simulink model "ImplantationCmd_LQI"  (R2022b)
settings: Solver=FixedStepDiscrete  StartTime=0.0  StopTime=60  FixedStep=Te1  MaxStep=0.001  RelTol=1e-3
values from neighbouring files (symbols this model uses):
  K_lqi = lqr(Apa,Bpa,Q_lqi,R_lqi)    [code.m]
  Kfi = 4.77    [code.m]
  Ki = 5    [code.m]
  Komga = 0.02    [code.m]
  Kteta = 0.875    [code.m]
  r = 0.022    [Validation_param_pend.m]    (also in code.m)
  Te1 = 0.100    (= 0.1)    [code.m]    (also in matlab.mat = 0)
undefined symbols (not defined in the file or in its folder): DiscIntNeverNeededParam, National_Instruments, PCI, pin
libraries: sldrtlib x3, simulink_extras x1
settings Model: SimulationMode=external  ExtModeTrigDuration=60000  Creator=Beauvois  LastModifiedBy=Pedro
settings SolverCC: AlgebraicLoopSolver=TrustRegion
settings DataIOCC: ReturnWorkspaceOutputs=off
settings DebuggingCC: UnconnectedInputMsg=warning  UnconnectedOutputMsg=warning  UnconnectedLineMsg=warning  SFMachineParentedDataDiag=warning  ArithmeticOperatorsInVariantConditions=warning
settings HardwareCC: ProdBitPerLong=64  ProdHWDeviceType=Intel->x86-64 (Linux 64)
settings ModelReferenceCC: EnableRefExpFcnMdlSchedulingChecks=on
settings SFSimCC: SimUseLocalCustomCode=off  CustomCodeUndefinedFunction=UseInterfaceOnly
settings RTWCC: Description=Simulink Desktop Real-Time  SystemTargetFile=sldrt.tlc  TemplateMakefile=sldrt.tmf  RTWUseLocalCustomCode=off  RTWCompilerOptimization=on
settings CodeAppCC: MaxIdLength=95
settings SimulinkDesktopRealTimeCC: TargetLibSuffix=_sldrt.a  TargetPreCompLibLocation=C:\Program Files\MATLAB\R2022b\toolbox\sldrt\lib\win64

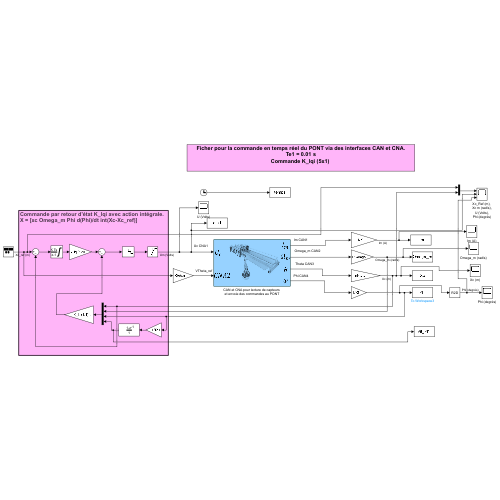
[thumbnail: Simulink's stored preview of the top-level diagram]
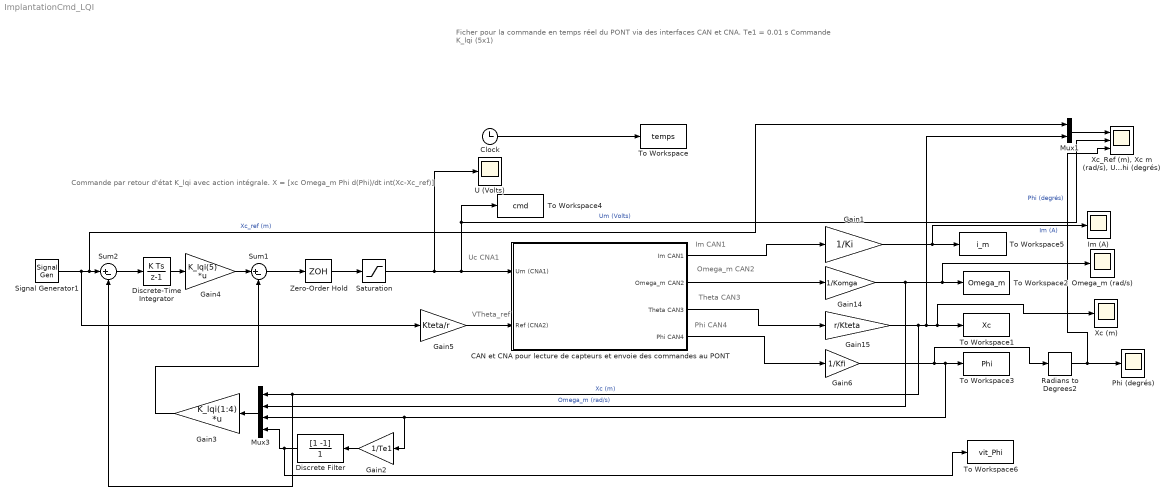
== system ImplantationCmd_LQI ==
  note: Commande par retour d'état K_lqi avec action intégrale.
      | X = [xc Omega_m Phi d(Phi)/dt int(Xc-Xc_ref)]
  note: Im CAN1
  note: Omega_m CAN2
  note: Theta CAN3
  note: Phi CAN4
  note: Uc CNA1
  note: VTheta_ref
  note: Ficher pour la commande en temps réel du PONT via des interfaces CAN et CNA.
      | Te1 = 0.01 s
      | Commande K_lqi (5x1)
  CAN et CNA pour lecture de capteurs et envoie des commandes au PONT : Subsystem
      mask Display: image('$imagefile'); % Use "Edit Image" on toolstrip to change.
  Clock : Clock
  Discrete Filter : DiscreteFilter  Numerator=[1 -1]  Denominator=1  SampleTime=Te1
  Discrete-Time Integrator : DiscreteIntegrator  SampleTime=Te1  LimitOutput=on  UpperSaturationLimit=1  LowerSaturationLimit=-1  ICPrevOutput=DiscIntNeverNeededParam  ICPrevScaledInput=DiscIntNeverNeededParam
  Gain1 : Gain  Gain=1/Ki
  Gain14 : Gain  Gain=1/Komga
  Gain15 : Gain  Gain=r/Kteta
  Gain2 : Gain  Gain=1/Te1
  Gain3 : Gain  Gain=K_lqi(1:4)  Multiplication=Matrix(K*u)
  Gain4 : Gain  Gain=K_lqi(5)  Multiplication=Matrix(K*u)
  Gain5 : Gain  Gain=Kteta/r
  Gain6 : Gain  Gain=1/Kfi
  Im (A) : Scope
  Mux1 : Mux  Inputs=2
  Mux3 : Mux
  Omega_m (rad/s) : Scope
  Phi (degrés) : Scope
  Radians to Degrees2 : simulink_extras/Transformations/Radians to Degrees
  Saturation : Saturate  UpperLimit=9.99  LowerLimit=-9.99
  Signal Generator1 : SignalGenerator  WaveForm=square  Amplitude=0.15  Frequency=0.05
  Sum1 : Sum  Inputs=|+-
  Sum2 : Sum  Inputs=|+-
  To Workspace : ToWorkspace  VariableName=temps  SampleTime=-1
  To Workspace1 : ToWorkspace  VariableName=Xc  SampleTime=-1
  To Workspace2 : ToWorkspace  VariableName=Omega_m  SampleTime=-1
  To Workspace3 : ToWorkspace  VariableName=Phi  SampleTime=-1
  To Workspace4 : ToWorkspace  VariableName=cmd  SampleTime=-1
  To Workspace5 : ToWorkspace  VariableName=i_m  SampleTime=-1
  To Workspace6 : ToWorkspace  VariableName=vit_Phi  SampleTime=-1
  U (Volts) : Scope
  Xc (m) : Scope
  "Xc_Ref (m), Xc m (rad/s), U (Volts), Phi (degrés)" : Scope  NumInputPorts=3
  Zero-Order Hold : ZeroOrderHold  SampleTime=Te1
  wires:
  Gain14/1 -> Mux3/2, To Workspace2/1, Omega_m (rad/s)/1  "Omega_m (rad/s)"
  Saturation/1 -> U (Volts)/1, CAN et CNA pour lecture de capteurs et envoie des commandes au PONT/1(Um (CNA1)), To Workspace4/1, "Xc_Ref (m), Xc m (rad/s), U (Volts), Phi (degrés)"/2  "Um (Volts)"
  Gain15/1 -> Mux3/1, Sum2/2, Mux1/2, Xc (m)/1, To Workspace1/1  "Xc (m)"
  Gain6/1 -> Gain2/1, Mux3/3, To Workspace3/1, Radians to Degrees2/1
  Radians to Degrees2/1 -> "Xc_Ref (m), Xc m (rad/s), U (Volts), Phi (degrés)"/3, Phi (degrés)/1  "Phi (degrés)"
  Clock/1 -> To Workspace/1
  Gain1/1 -> Im (A)/1, To Workspace5/1  "Im (A)"
  CAN et CNA pour lecture de capteurs et envoie des commandes au PONT/1(Im CAN1) -> Gain1/1
  CAN et CNA pour lecture de capteurs et envoie des commandes au PONT/2(Omega_m CAN2) -> Gain14/1
  CAN et CNA pour lecture de capteurs et envoie des commandes au PONT/3(Theta CAN3) -> Gain15/1
  CAN et CNA pour lecture de capteurs et envoie des commandes au PONT/4(Phi CAN4) -> Gain6/1
  Signal Generator1/1 -> Mux1/1, Sum2/1, Gain5/1  "Xc_ref (m)"
  Gain4/1 -> Sum1/1
  Zero-Order Hold/1 -> Saturation/1
  Sum1/1 -> Zero-Order Hold/1
  Gain3/1 -> Sum1/2
  Mux3/1 -> Gain3/1
  Discrete Filter/1 -> To Workspace6/1, Mux3/4
  Gain2/1 -> Discrete Filter/1
  Gain5/1 -> CAN et CNA pour lecture de capteurs et envoie des commandes au PONT/2(Ref (CNA2))
  Discrete-Time Integrator/1 -> Gain4/1
  Sum2/1 -> Discrete-Time Integrator/1
  Mux1/1 -> "Xc_Ref (m), Xc m (rad/s), U (Volts), Phi (degrés)"/1

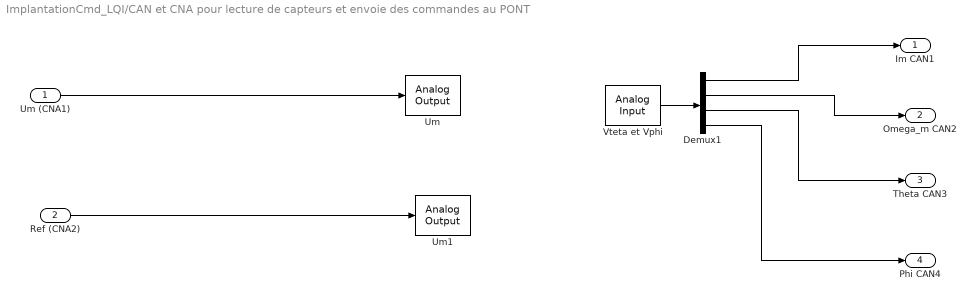
== system ImplantationCmd_LQI/CAN et CNA pour lecture de capteurs et envoie des commandes au PONT ==
  Um (CNA1) : Inport
  Ref (CNA2) : Inport  Port=2
  Demux1 : Demux
  Um : sldrtlib/Analog Output  SampleTime=Te1  MaxMissedTicks=10  ShowMissedTicks=off  YieldWhenWaiting=off  DrvName=National_Instruments/PCI-6221_37-pin  DrvAddress=4294967295  DrvOptions=[0 0 0 0 0]  Channels=1  RangeMode=1  VoltRange=1  InitialValue=0  FinalValue=0
      settings: AttributesFormatString=National Instruments\nPCI-6221 37-pin [auto]
  Um1 : sldrtlib/Analog Output  SampleTime=Te1  MaxMissedTicks=10  ShowMissedTicks=off  YieldWhenWaiting=off  DrvName=National_Instruments/PCI-6221_37-pin  DrvAddress=4294967295  DrvOptions=[0 0 0 0 0]  Channels=2  RangeMode=1  VoltRange=1  InitialValue=0  FinalValue=0
      settings: AttributesFormatString=National Instruments\nPCI-6221 37-pin [auto]
  Vteta et Vphi : sldrtlib/Analog Input  SampleTime=Te1  MaxMissedTicks=10  ShowMissedTicks=off  YieldWhenWaiting=off  DrvName=National_Instruments/PCI-6221_37-pin  DrvAddress=4294967295  DrvOptions=[0 0 0 0 0]  Channels=[1 2 3 4]  RangeMode=1  VoltRange=1  DataType=1
      settings: AttributesFormatString=National Instruments\nPCI-6221 37-pin [auto]
  Im CAN1 : Outport
  Omega_m CAN2 : Outport  Port=2
  Theta CAN3 : Outport  Port=3
  Phi CAN4 : Outport  Port=4
  wires:
  Vteta et Vphi/1 -> Demux1/1
  Um (CNA1)/1 -> Um/1
  Demux1/1 -> Im CAN1/1
  Demux1/4 -> Phi CAN4/1
  Demux1/3 -> Theta CAN3/1
  Demux1/2 -> Omega_m CAN2/1
  Ref (CNA2)/1 -> Um1/1
